simulink model "slipControl"  (R2025b)
settings: Solver=VariableStepAuto  StartTime=0.0  StopTime=10.0  RelTol=1e-3
model workspace (MAT data in the model file):
  Jw = 1
libraries: slpidlib x2
settings Model: Creator=zinga  LastModifiedBy=zinga

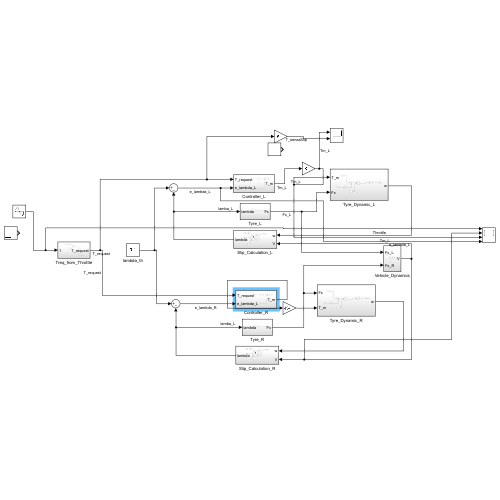
[thumbnail: Simulink's stored preview of the top-level diagram]
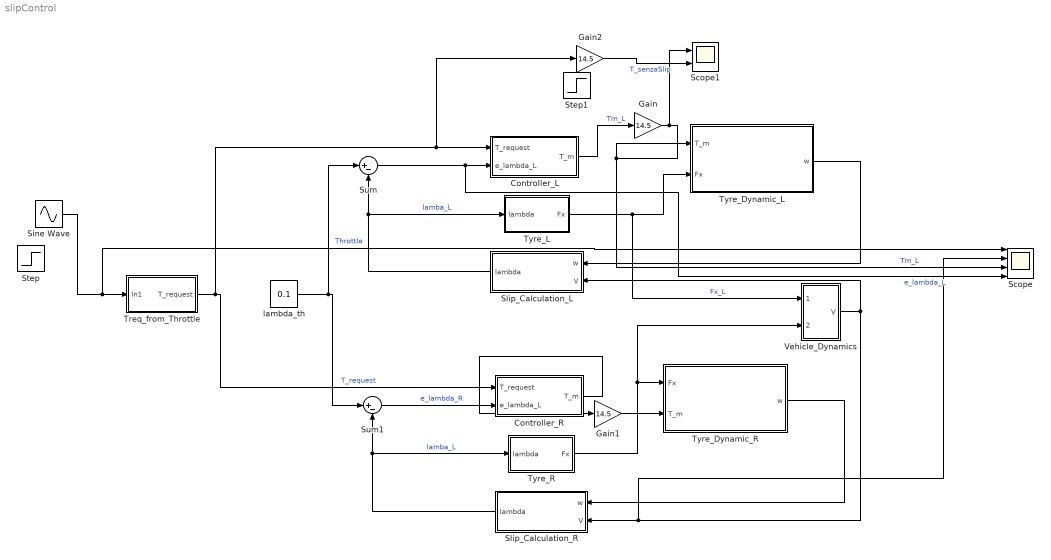
== system slipControl ==
  Controller_L : Subsystem
  Controller_R : Subsystem
  Gain : Gain  Gain=14.5
  Gain1 : Gain  Gain=14.5
  Gain2 : Gain  Gain=14.5
  Scope : Scope  NumInputPorts=4
      settings: ActiveDisplayYMinimum=-37.341126922230764  ActiveDisplayYMaximum=336.07014230007695
  Scope1 : Scope  NumInputPorts=2
      settings: ActiveDisplayYMinimum=39.309851400419141  ActiveDisplayYMaximum=333.9655720666201
  Sine Wave : Sin  Amplitude=100  Frequency=0.1  Phase=pi/2  SampleTime=0.05
  Slip_Calculation_L : Subsystem
  Slip_Calculation_R : Subsystem
  Step : Step  After=100  SampleTime=0
  Step1 : Step  After=21  SampleTime=0
  Sum : Sum  Inputs=|+-
  Sum1 : Sum  Inputs=|+-
  Treq_from_Throttle : Subsystem
  Tyre_Dynamic_L : Subsystem
  Tyre_Dynamic_R : Subsystem
  Tyre_L : Subsystem
  Tyre_R : Subsystem
  Vehicle_Dynamics : Subsystem
  lambda_th : Constant  Value=0.1
  wires:
  Slip_Calculation_L/1(lambda) -> Tyre_L/1(lambda), Sum/2  "lamba_L"
  Sine Wave/1 -> Scope/1, Treq_from_Throttle/1(In1)  "Throttle"
  Sum/1 -> Scope/4, Controller_L/2(e_lambda_L)  "e_lambda_L"
  Treq_from_Throttle/1(T_request) -> Controller_R/1(T_request), Gain2/1, Controller_L/1(T_request)  "T_request"
  Gain/1 -> Tyre_Dynamic_L/1(T_m), Scope/3, Scope1/1  "Tm_L"
  Tyre_L/1(Fx) -> Tyre_Dynamic_L/2(Fx), Vehicle_Dynamics/1(Fx_L)  "Fx_L"
  Tyre_Dynamic_L/1(w) -> Slip_Calculation_L/1(w)
  Slip_Calculation_R/1(lambda) -> Tyre_R/1(lambda), Sum1/2  "lamba_L"
  Vehicle_Dynamics/1(V) -> Scope/2, Slip_Calculation_R/2(V), Slip_Calculation_L/2(V)
  Tyre_Dynamic_R/1(w) -> Slip_Calculation_R/1(w)
  Tyre_R/1(Fx) -> Vehicle_Dynamics/2(Fx_R), Tyre_Dynamic_R/1(Fx)
  lambda_th/1 -> Sum1/1, Sum/1
  Sum1/1 -> Controller_R/2(e_lambda_L)  "e_lambda_R"
  Gain1/1 -> Tyre_Dynamic_R/2(T_m)
  Controller_L/1(T_m) -> Gain/1  "Tm_L"
  Controller_R/1(T_m) -> Gain1/1
  Gain2/1 -> Scope1/2  "T_senzaSlip"

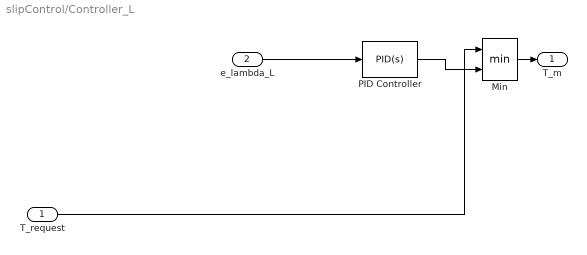
== system slipControl/Controller_L ==
  T_request : Inport
  e_lambda_L : Inport  Port=2
  Min : MinMax  Inputs=2
  PID Controller : slpidlib/PID Controller  Controller=PID  Form=Parallel  TimeDomain=Continuous-time  UseExternalTs=off  SampleTime=-1  IntegratorMethod=Forward Euler  FilterMethod=Forward Euler  ControllerParametersSource=internal  P=50  I=100  UseKiTs=off  D=0  UseExternalDerivativeSource=off  N=100  UseFilter=on  TunerSelectOption=Transfer Function Based (PID Tuner App)  InitialConditionSource=internal  InitialConditionForIntegrator=0  InitialConditionForFilter=0  DifferentiatorICPrevScaledInput=0  ExternalReset=none  TrackingMode=off  Kt=1  LimitOutput=on  SatLimitsSource=internal  UpperSaturationLimit=21  LowerSaturationLimit=0  LinearizeAsGain=on  AntiWindupMode=clamping  Kb=1  LimitIntegrator=off  UpperIntegratorSaturationLimit=inf  LowerIntegratorSaturationLimit=-inf  POutMin=[]  POutMax=[]  IOutMin=[]  IOutMax=[]  DOutMin=[]  DOutMax=[]  NOutMin=[]  NOutMax=[]  SumOutMin=[]  SumOutMax=[]  SaturationOutMin=[]  SaturationOutMax=[]  PParamMin=[]  PParamMax=[]  IParamMin=[]  IParamMax=[]  DParamMin=[]  DParamMax=[]  NParamMin=[]  NParamMax=[]  KbParamMin=[]  KbParamMax=[]  KtParamMin=[]  KtParamMax=[]  KbOutMin=[]  KbOutMax=[]  KtOutMin=[]  KtOutMax=[]  IntegratorOutMin=[]  IntegratorOutMax=[]  FilterOutMin=[]  FilterOutMax=[]  SumI1OutMin=[]  SumI1OutMax=[]  SumI2OutMin=[]  SumI2OutMax=[]  SumI3OutMin=[]  SumI3OutMax=[]  SumI4OutMin=[]  SumI4OutMax=[]  SumDOutMin=[]  SumDOutMax=[]  DifferentiatorOutMin=[]  DifferentiatorOutMax=[]  FilterDiffOutCoefMin=[]  FilterDiffOutCoefMax=[]  ReciprocalOutMin=[]  ReciprocalOutMax=[]  SumDenOutMin=[]  SumDenOutMax=[]  SumNumOutMin=[]  SumNumOutMax=[]  DivideOutMin=[]  DivideOutMax=[]  UdiffTsProdOutMin=[]  UdiffTsProdOutMax=[]  NTsProdOutMin=[]  NTsProdOutMax=[]  UintegralTsProdOutMin=[]  UintegralTsProdOutMax=[]  UngainTsProdOutMin=[]  UngainTsProdOutMax=[]  ClampingZeroOutDataTypeStr=Inherit: Inherit via back propagation  ClampingZeroOutMin=[]  ClampingZeroOutMax=[]  FilterDenConstantOutDataTypeStr=Inherit: Inherit via back propagation  FilterDenConstantOutMin=[]  FilterDenConstantOutMax=[]  PCopyOutDataTypeStr=Inherit: Inherit via back propagation  PCopyOutMin=[]  PCopyOutMax=[]  NCopyOutDataTypeStr=Inherit: Inherit via back propagation  NCopyOutMin=[]  NCopyOutMax=[]  IntegratorContinuousStateAttributes=''  IntegratorStateMustResolveToSignalObject=off  IntegratorRTWStateStorageClass=Auto  FilterContinuousStateAttributes=''  FilterStateMustResolveToSignalObject=off  FilterRTWStateStorageClass=Auto  ParallelPVariant=InternalParameters  IdealPVariant=Disabled  IVariant=InternalParameters  DVariant=InternalParameters  IntegratorVariant=Continuous  SatVariant=Enabled  AWVariant=ContClampingParallel  PCopyVariant=Disabled  TRVariant=Disabled  FdbkBlocksVariant=Forward  IdealPFdbkVariant=Disabled  SatFdbkVariant=Disabled  DerivativeFilterVariant=ContFilter  NVariant=InternalParameters  NCopyVariant=Disabled  FilterICVariant=InternalICsFilter  IntegratorICVariant=InternalICs  ExternalResetVariant=Disabled  TRSumVariant=Passthrough  SumFdbkVariant=Disabled  SumVariant=Sum_PID  TsampFilterVariant=InternalTs  TsampNgainVariant=Passthrough  TsampIntegralVariant=Disabled_SignalSpec  ExternalSaturationOutDataTypeStr=Inherit: Same as second input  DerivativeSourceVariant=ErrorSignal  PreIntVariant=InternalPreInt
  T_m : Outport
  wires:
  Min/1 -> T_m/1
  PID Controller/1 -> Min/2
  T_request/1 -> Min/1
  e_lambda_L/1 -> PID Controller/1

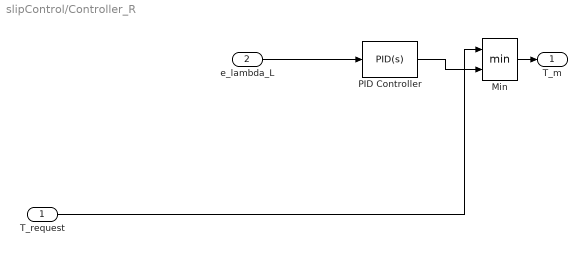
== system slipControl/Controller_R ==
  T_request : Inport
  e_lambda_L : Inport  Port=2
  Min : MinMax  Inputs=2
  PID Controller : slpidlib/PID Controller  Controller=PID  Form=Parallel  TimeDomain=Continuous-time  UseExternalTs=off  SampleTime=-1  IntegratorMethod=Forward Euler  FilterMethod=Forward Euler  ControllerParametersSource=internal  P=50  I=100  UseKiTs=off  D=0  UseExternalDerivativeSource=off  N=100  UseFilter=on  TunerSelectOption=Transfer Function Based (PID Tuner App)  InitialConditionSource=internal  InitialConditionForIntegrator=0  InitialConditionForFilter=0  DifferentiatorICPrevScaledInput=0  ExternalReset=none  TrackingMode=off  Kt=1  LimitOutput=on  SatLimitsSource=internal  UpperSaturationLimit=21  LowerSaturationLimit=0  LinearizeAsGain=on  AntiWindupMode=clamping  Kb=1  LimitIntegrator=off  UpperIntegratorSaturationLimit=inf  LowerIntegratorSaturationLimit=-inf  POutMin=[]  POutMax=[]  IOutMin=[]  IOutMax=[]  DOutMin=[]  DOutMax=[]  NOutMin=[]  NOutMax=[]  SumOutMin=[]  SumOutMax=[]  SaturationOutMin=[]  SaturationOutMax=[]  PParamMin=[]  PParamMax=[]  IParamMin=[]  IParamMax=[]  DParamMin=[]  DParamMax=[]  NParamMin=[]  NParamMax=[]  KbParamMin=[]  KbParamMax=[]  KtParamMin=[]  KtParamMax=[]  KbOutMin=[]  KbOutMax=[]  KtOutMin=[]  KtOutMax=[]  IntegratorOutMin=[]  IntegratorOutMax=[]  FilterOutMin=[]  FilterOutMax=[]  SumI1OutMin=[]  SumI1OutMax=[]  SumI2OutMin=[]  SumI2OutMax=[]  SumI3OutMin=[]  SumI3OutMax=[]  SumI4OutMin=[]  SumI4OutMax=[]  SumDOutMin=[]  SumDOutMax=[]  DifferentiatorOutMin=[]  DifferentiatorOutMax=[]  FilterDiffOutCoefMin=[]  FilterDiffOutCoefMax=[]  ReciprocalOutMin=[]  ReciprocalOutMax=[]  SumDenOutMin=[]  SumDenOutMax=[]  SumNumOutMin=[]  SumNumOutMax=[]  DivideOutMin=[]  DivideOutMax=[]  UdiffTsProdOutMin=[]  UdiffTsProdOutMax=[]  NTsProdOutMin=[]  NTsProdOutMax=[]  UintegralTsProdOutMin=[]  UintegralTsProdOutMax=[]  UngainTsProdOutMin=[]  UngainTsProdOutMax=[]  ClampingZeroOutDataTypeStr=Inherit: Inherit via back propagation  ClampingZeroOutMin=[]  ClampingZeroOutMax=[]  FilterDenConstantOutDataTypeStr=Inherit: Inherit via back propagation  FilterDenConstantOutMin=[]  FilterDenConstantOutMax=[]  PCopyOutDataTypeStr=Inherit: Inherit via back propagation  PCopyOutMin=[]  PCopyOutMax=[]  NCopyOutDataTypeStr=Inherit: Inherit via back propagation  NCopyOutMin=[]  NCopyOutMax=[]  IntegratorContinuousStateAttributes=''  IntegratorStateMustResolveToSignalObject=off  IntegratorRTWStateStorageClass=Auto  FilterContinuousStateAttributes=''  FilterStateMustResolveToSignalObject=off  FilterRTWStateStorageClass=Auto  ParallelPVariant=InternalParameters  IdealPVariant=Disabled  IVariant=InternalParameters  DVariant=InternalParameters  IntegratorVariant=Continuous  SatVariant=Enabled  AWVariant=ContClampingParallel  PCopyVariant=Disabled  TRVariant=Disabled  FdbkBlocksVariant=Forward  IdealPFdbkVariant=Disabled  SatFdbkVariant=Disabled  DerivativeFilterVariant=ContFilter  NVariant=InternalParameters  NCopyVariant=Disabled  FilterICVariant=InternalICsFilter  IntegratorICVariant=InternalICs  ExternalResetVariant=Disabled  TRSumVariant=Passthrough  SumFdbkVariant=Disabled  SumVariant=Sum_PID  TsampFilterVariant=InternalTs  TsampNgainVariant=Passthrough  TsampIntegralVariant=Disabled_SignalSpec  ExternalSaturationOutDataTypeStr=Inherit: Same as second input  DerivativeSourceVariant=ErrorSignal  PreIntVariant=InternalPreInt
  T_m : Outport
  wires:
  Min/1 -> T_m/1
  PID Controller/1 -> Min/2
  T_request/1 -> Min/1
  e_lambda_L/1 -> PID Controller/1

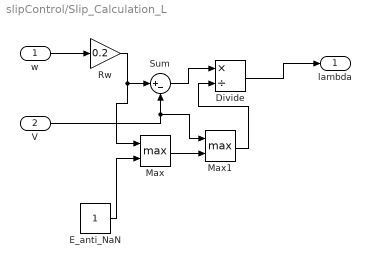
== system slipControl/Slip_Calculation_L ==
  w : Inport
  V : Inport  Port=2
  Divide : Product  Inputs=*/
  E_anti_NaN : Constant
  Max : MinMax  Function=max  Inputs=2
  Max1 : MinMax  Function=max  Inputs=2
  Rw : Gain  Gain=0.2
  Sum : Sum  Inputs=|+-
  lambda : Outport
  wires:
  w/1 -> Rw/1
  V/1 -> Max1/1, Sum/2
  Rw/1 -> Max/1, Sum/1
  Sum/1 -> Divide/1
  E_anti_NaN/1 -> Max/2
  Max/1 -> Max1/2
  Max1/1 -> Divide/2
  Divide/1 -> lambda/1

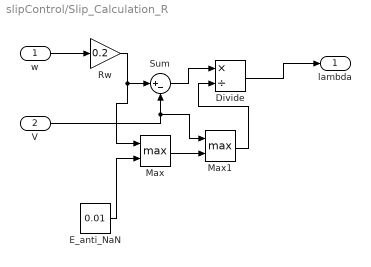
== system slipControl/Slip_Calculation_R ==
  w : Inport
  V : Inport  Port=2
  Divide : Product  Inputs=*/
  E_anti_NaN : Constant  Value=0.01
  Max : MinMax  Function=max  Inputs=2
  Max1 : MinMax  Function=max  Inputs=2
  Rw : Gain  Gain=0.2
  Sum : Sum  Inputs=|+-
  lambda : Outport
  wires:
  w/1 -> Rw/1
  V/1 -> Max1/1, Sum/2
  Rw/1 -> Max/1, Sum/1
  Sum/1 -> Divide/1
  E_anti_NaN/1 -> Max/2
  Max/1 -> Max1/2
  Max1/1 -> Divide/2
  Divide/1 -> lambda/1

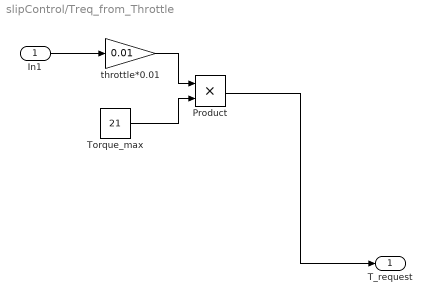
== system slipControl/Treq_from_Throttle ==
  In1 : Inport
  Product : Product
  Torque_max : Constant  Value=21
  throttle*0.01 : Gain  Gain=0.01
  T_request : Outport
  wires:
  throttle*0.01/1 -> Product/1
  In1/1 -> throttle*0.01/1
  Torque_max/1 -> Product/2
  Product/1 -> T_request/1

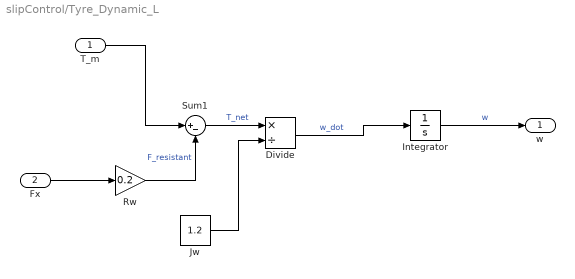
== system slipControl/Tyre_Dynamic_L ==
  T_m : Inport
  Fx : Inport  Port=2
  Divide : Product  Inputs=*/
  Integrator : Integrator
  Jw : Constant  Value=1.2
  Rw : Gain  Gain=0.2
  Sum1 : Sum  Inputs=|+-
  w : Outport
  wires:
  T_m/1 -> Sum1/1
  Divide/1 -> Integrator/1  "w_dot"
  Rw/1 -> Sum1/2  "F_resistant"
  Fx/1 -> Rw/1
  Sum1/1 -> Divide/1  "T_net"
  Jw/1 -> Divide/2
  Integrator/1 -> w/1  "w"

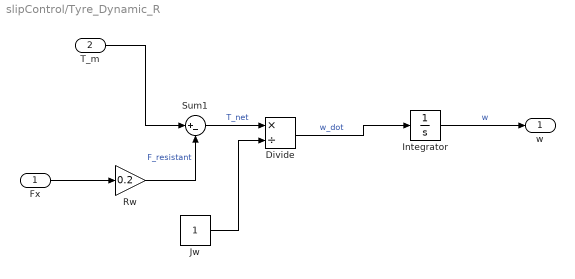
== system slipControl/Tyre_Dynamic_R ==
  Fx : Inport
  T_m : Inport  Port=2
  Divide : Product  Inputs=*/
  Integrator : Integrator
  Jw : Constant
  Rw : Gain  Gain=0.2
  Sum1 : Sum  Inputs=|+-
  w : Outport
  wires:
  T_m/1 -> Sum1/1
  Divide/1 -> Integrator/1  "w_dot"
  Rw/1 -> Sum1/2  "F_resistant"
  Fx/1 -> Rw/1
  Sum1/1 -> Divide/1  "T_net"
  Jw/1 -> Divide/2
  Integrator/1 -> w/1  "w"

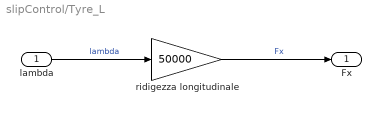
== system slipControl/Tyre_L ==
  lambda : Inport
  ridigezza longitudinale : Gain  Gain=50000
  Fx : Outport
  wires:
  ridigezza longitudinale/1 -> Fx/1  "Fx"
  lambda/1 -> ridigezza longitudinale/1  "lambda"

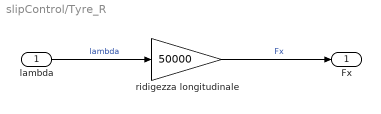
== system slipControl/Tyre_R ==
  lambda : Inport
  ridigezza longitudinale : Gain  Gain=50000
  Fx : Outport
  wires:
  ridigezza longitudinale/1 -> Fx/1  "Fx"
  lambda/1 -> ridigezza longitudinale/1  "lambda"

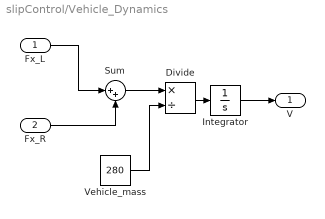
== system slipControl/Vehicle_Dynamics ==
  Fx_L : Inport
  Fx_R : Inport  Port=2
  Divide : Product  Inputs=*/
  Integrator : Integrator
  Sum : Sum  Inputs=|++
  Vehicle_mass : Constant  Value=280
  V : Outport
  wires:
  Fx_R/1 -> Sum/2
  Fx_L/1 -> Sum/1
  Integrator/1 -> V/1
  Vehicle_mass/1 -> Divide/2
  Sum/1 -> Divide/1
  Divide/1 -> Integrator/1
